simulink model "Multirotor_NMPC_Updated"  (R2021a)
settings: Solver=ode4  StartTime=0.0  StopTime=20  FixedStep=0.001  RelTol=1e-3
libraries: mpclib x1
settings Model: Creator=Hameed  LastModifiedBy=Hameed

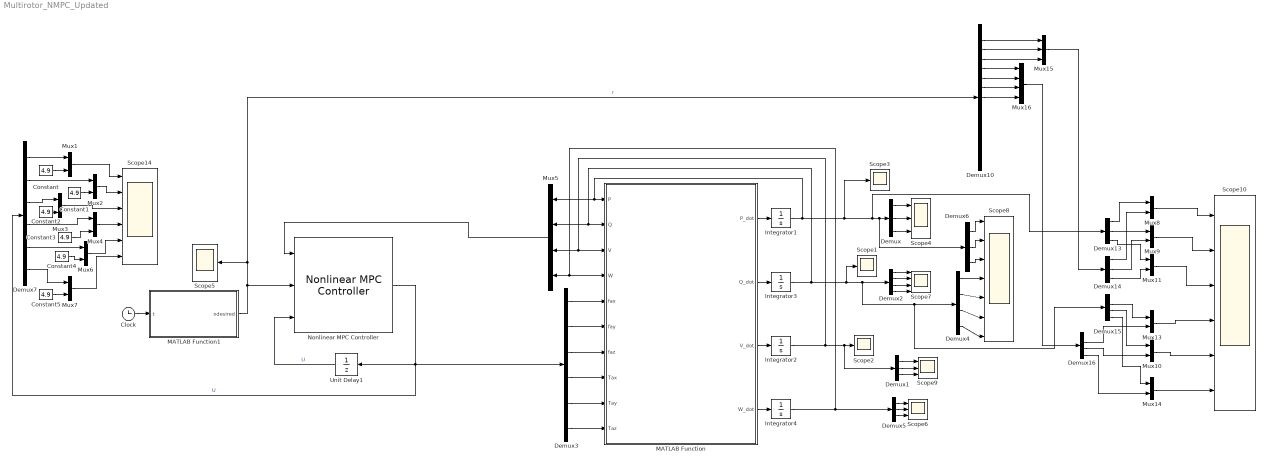
== system Multirotor_NMPC_Updated ==
  Clock : Clock
  Constant{,1..5} (6 alike) : Constant  Value=4.9
  Demux{,1,5..6,13..14} (6 alike) : Demux  Outputs=3
  Demux10 : Demux  Outputs=13
  Demux{2,4,15..16} (4 alike) : Demux
  Demux3 : Demux  Outputs=6
  Demux7 : Demux  Outputs=6
  Integrator1 : Integrator  InitialCondition=[7;-10;0]
  Integrator2 : Integrator  InitialCondition=[0;0;0]
  Integrator3 : Integrator  InitialCondition=[0;0;0;0]
  Integrator4 : Integrator  InitialCondition=[0;0;0]
  MATLAB Function : MATLAB Function  TreatAsAtomicUnit=on
  MATLAB Function1 : MATLAB Function  TreatAsAtomicUnit=on
  Mux{1..4,6..11,13..14} (12 alike) : Mux  Inputs=2
  Mux15 : Mux  Inputs=3
  Mux16 : Mux
  Mux5 : Mux
  Nonlinear MPC Controller : mpclib/Nonlinear MPC Controller  SCDEnableBlockLinearizationSpecification=on  nlmpcobj=nlobj12  UseObjectTs=on  UseMEX=off  md_enabled=off  mvtarget_enabled=off  param_enabled=off  cost_enabled=off  mvseq_enabled=off  stateseq_enabled=off  ovseq_enabled=off  slack_enabled=off  status_enabled=off  ov_min=off  ov_max=off  mv_min=off  mv_max=off  mvrate_min=off  mvrate_max=off  state_min=off  state_max=off  ov_weight=off  mv_weight=off  mvrate_weight=off  ecr_weight=off  nlp_initialize=off
  Scope{1..3,5} (4 alike) : Scope
  Scope10 : Scope  NumInputPorts=6
  Scope14 : Scope  NumInputPorts=6
  Scope4 : Scope  NumInputPorts=3
  Scope6 : Scope  NumInputPorts=3
  Scope7 : Scope  NumInputPorts=4
  Scope8 : Scope  NumInputPorts=7
  Scope9 : Scope  NumInputPorts=3
  Unit Delay1 : UnitDelay  InitialCondition=[4.9;4.9;4.9;4.9;4.9;4.9]  SampleTime=0.1  HasFrameUpgradeWarning=on
  wires:
  Nonlinear MPC Controller/1 -> Unit Delay1/1, Demux7/1, Demux3/1  "U"
  MATLAB Function1/1(xdesired) -> Demux10/1, Scope5/1, Nonlinear MPC Controller/2  "r"
  Clock/1 -> MATLAB Function1/1(t)
  MATLAB Function/3(V_dot) -> Integrator2/1
  Demux3/4 -> MATLAB Function/8(Tax)
  Demux3/6 -> MATLAB Function/10(Taz)
  MATLAB Function/4(W_dot) -> Integrator4/1
  Demux3/3 -> MATLAB Function/7(faz)
  MATLAB Function/1(P_dot) -> Integrator1/1
  MATLAB Function/2(Q_dot) -> Integrator3/1
  Demux3/2 -> MATLAB Function/6(fay)
  Demux3/1 -> MATLAB Function/5(fax)
  Demux3/5 -> MATLAB Function/9(Tay)
  Mux5/1 -> Nonlinear MPC Controller/1
  Demux2/2 -> Scope7/2
  Integrator2/1 -> MATLAB Function/3(V), Mux5/3, Demux1/1, Scope2/1
  Demux/1 -> Scope4/1
  Demux1/3 -> Scope9/3
  Demux/2 -> Scope4/2
  Demux5/3 -> Scope6/3
  Demux2/1 -> Scope7/1
  Demux5/2 -> Scope6/2
  Demux/3 -> Scope4/3
  Demux2/4 -> Scope7/4
  Demux1/1 -> Scope9/1
  Demux1/2 -> Scope9/2
  Demux5/1 -> Scope6/1
  Integrator4/1 -> MATLAB Function/4(W), Mux5/4, Demux5/1
  Demux2/3 -> Scope7/3
  Demux4/1 -> Scope8/4
  Demux4/2 -> Scope8/5
  Demux4/3 -> Scope8/6
  Demux4/4 -> Scope8/7
  Demux6/1 -> Scope8/1
  Demux6/2 -> Scope8/2
  Demux6/3 -> Scope8/3
  Mux3/1 -> Scope14/3
  Constant1/1 -> Mux2/2
  Unit Delay1/1 -> Nonlinear MPC Controller/3  "U"
  Constant/1 -> Mux1/2
  Mux4/1 -> Scope14/4
  Demux7/3 -> Mux3/1
  Constant2/1 -> Mux3/2
  Mux2/1 -> Scope14/2
  Mux1/1 -> Scope14/1
  Demux7/4 -> Mux4/1
  Constant3/1 -> Mux4/2
  Demux7/2 -> Mux2/1
  Demux7/1 -> Mux1/1
  Demux7/5 -> Mux6/1
  Demux7/6 -> Mux7/1
  Constant4/1 -> Mux6/2
  Constant5/1 -> Mux7/2
  Mux6/1 -> Scope14/5
  Mux7/1 -> Scope14/6
  Integrator1/1 -> Mux5/1, MATLAB Function/1(P), Scope3/1, Demux13/1, Demux6/1, Demux/1
  Demux16/3 -> Mux10/2
  Demux14/3 -> Mux11/2
  Mux11/1 -> Scope10/3
  Demux14/1 -> Mux8/2
  Demux15/3 -> Mux10/1
  Integrator3/1 -> Mux5/2, MATLAB Function/2(Q), Scope1/1, Demux15/1, Demux4/1, Demux2/1
  Demux13/2 -> Mux9/1
  Demux14/2 -> Mux9/2
  Demux13/3 -> Mux11/1
  Demux16/2 -> Mux13/2
  Demux15/2 -> Mux13/1
  Demux13/1 -> Mux8/1
  Mux9/1 -> Scope10/2
  Mux8/1 -> Scope10/1
  Demux10/1 -> Mux15/1
  Demux10/2 -> Mux15/2
  Demux10/3 -> Mux15/3
  Mux15/1 -> Demux14/1
  Demux10/4 -> Mux16/1
  Demux10/5 -> Mux16/2
  Demux10/6 -> Mux16/3
  Demux10/7 -> Mux16/4
  Mux16/1 -> Demux16/1
  Demux16/4 -> Mux14/2
  Demux15/4 -> Mux14/1
  Mux13/1 -> Scope10/4
  Mux10/1 -> Scope10/5
  Mux14/1 -> Scope10/6

== matlab function Multirotor_NMPC_Updated/MATLAB Function1 ==
  data: t input; xdesired output
function xdesired   = MultirotorReferenceTrajectory( t )
% This function generates reference signal for nonlinear MPC controller
% used in the quadrotor path following example.

% Copyright 2019 The MathWorks, Inc.

%#codegen
% P(1) =6*sin(t/3);
% P(2) = -6*sin(t/3).*cos(t/3);
% P(3)= 6*cos(t/3);
% %z = 10+zeros(1,length(t));
% Q(1)= zeros(1,length(t));
% Q(2)= zeros(1,length(t));
% Q(3) = zeros(1,length(t));
% Q(4) = zeros(1,length(t));
% 
% V(1)= zeros(1,length(t));
% V(2) = zeros(1,length(t));
% V(3) = zeros(1,length(t));
% 
% W(1) = zeros(1,length(t));
% W(2) = zeros(1,length(t));
% W(3) = zeros(1,length(t));


x =6*sin(t/3);
y = -6*sin(t/3).*cos(t/3);
z = 6*cos(t/3);
%z = 10+zeros(1,length(t));
qw = zeros(1,length(t));
phi = zeros(1,length(t));
theta = zeros(1,length(t));
psi = zeros(1,length(t));
% phi = pi/6*sin(t/3);
% theta = -pi/3*sin(t/3).*cos(t/3);
% psi = pi*ones(1,length(t));
xdot = zeros(1,length(t));
ydot = zeros(1,length(t));
zdot = zeros(1,length(t));
phidot = zeros(1,length(t));
thetadot = zeros(1,length(t));
psidot = zeros(1,length(t));

xdesired = [x;y;z;qw;phi;theta;psi;xdot;ydot;zdot;phidot;thetadot;psidot]';
%xdesired = [P(1);P(2);P(3);Q(1);Q(2);Q(3);Q(4);V(1);V(2);V(3);W(1);W(2);W(3)]';
end

== matlab function Multirotor_NMPC_Updated/MATLAB Function ==
  data: P input; Q input; P_dot output; Q_dot output; V input; W input; V_dot output; W_dot output; fax input; fay input; faz input; Tax input; Tay input; Taz input
function [P_dot,Q_dot,V_dot,W_dot]= fcn(P,Q,V,W,fax,fay,faz,Tax,Tay,Taz)
clc
m=5;

%%% phi=Q(2); % theta=Q(3); % psi=Q(4);

% Rz=[cos(psi) sin(psi) 0;-sin(psi)) cos(psi) 0;0 0 1];
% Rx=[1 0 0;0 cos(phi) sin(phi);0 -sin(phi) cos(phi)];
% Ry=[cos(theta) 0 -sin(theta);0 1 0;sin(theta) 0 cos(theta)];

Rz=[cos(Q(4)) sin(Q(4)) 0; -sin(Q(4)) cos(Q(4)) 0; 0 0 1];
Rx=[1 0 0; 0 cos(Q(2)) sin(Q(2)); 0 -sin(Q(2)) cos(Q(2))];
Ry=[cos(Q(3)) 0 -sin(Q(3)); 0 1 0; sin(Q(3)) 0 cos(Q(3))];

Rb=Rz*Ry*Rx;
Rs=[1 0 0;
    0 0 -1;
    0 1 0 ];

%Rs=[1 0 0;0 -1 0;0 0 -1];
%lambda=L;
L=0;
%L=1;
Rd=[1 0 0;
    0 1 0;
    0 0 1-L];

SL=Rs*Rd*transpose(Rs);

rT=[0.5;0;0];

Ixx=1;
Iyy=1;
Izz=1;
J=[Ixx 0 0;0 Iyy 0;0 0 Izz];

g=9.8;
dF=[0;0;0];
fc=[0;0;0];
rcom=[0;0;0];
dT=[0;0;0];

fa=[fax;fay;faz];
ta=[Tax;Tay;Taz];

ab=(m^-1)*((Rb*fa)+(L*fc)+dF)+[0;0;g];

% T=[0 -sin(Q(2)) cos(Q(2))*sin(Q(3));
% 0 cos(Q(2)) sin(Q(2))*sin(Q(3));
% 1 0 cos(Q(3))];

Sq=[0 -Q(4) Q(3);
    Q(4) 0 -Q(2);
    -Q(3) Q(2) 0];

eata_dot=[Q(2);Q(3);Q(4)]
%w=T*eata_dot;

h=J*W;
h1=transpose(Rb)*[0;0;m*g];
h2=L*transpose(Rb)*fc;

P_dot=SL*V;

Qw_dot=-1/2*[Q(2) Q(3) Q(4)]*W;
Qv_dot=1/2*(Q(1)*J-Sq)*W;

% Qw_dot=-1/2*[Q(2) Q(3) Q(4)]*W
% Qv_dot=1/2*(Q(1)*J-Sq)*W;
Q_dot=[Qw_dot;Qv_dot];

W_dot=(inv(J))*(ta-cross(W,h)+cross(rcom,h1)+cross(rT,h2)+dT);

V_dot=SL*((ab)+Rb*(cross(W_dot,rT)+(cross(W,cross(W,rT)))));
